simulink model "LKAS"  (R2018b)
settings: Solver=FixedStepDiscrete  StartTime=0.0  StopTime=10.0  FixedStep=0.01  RelTol=1e-3
InitFcn:
  | tmpVer = ver('MATLAB');
  | tmpVer = str2num(tmpVer.Version);
  | % -------------------------------------------------------------------
  | %  MATLAB file generated by Simulink.saveVars on 21-Nov-2019 10:06:14
  | %  MATLAB version: 7.13.0.564 (R2011b)
  | % -------------------------------------------------------------------
  | 
  | 
  | SInt16 = Simulink.AliasType;
  | SInt16.Description = 'Num';
  | if (tmpVer > 7.11)
  | 	SInt16.DataScope = 'Auto';
  | end
  | SInt16.HeaderFile = 'Rte_Type.h';
  | SInt16.BaseType = 'int16';
  | 
  | SInt32 = Simulink.AliasType;
  | SInt32.Description = 'Num';
  | if (tmpVer > 7.11)
  | 	SInt32.DataScope = 'Auto';
  | end
  | SInt32.HeaderFile = 'Rte_Type.h';
  | SInt32.BaseType = 'int32';
  | 
  | SInt8 = Simulink.AliasType;
  | SInt8.Description = 'Num';
  | if (tmpVer > 7.11)
  | 	SInt8.DataScope = 'Auto';
  | end
  | SInt8.HeaderFile = 'Rte_Type.h';
  | SInt8.BaseType = 'int8';
  | 
  | T_A_m2_1024_1_u32 = Simulink.NumericType;
  | T_A_m2_1024_1_u32.Description = 'm2 (square meters  (m2))';
  | if (tmpVer > 7.11)
  | 	T_A_m2_1024_1_u32.DataScope = 'Auto';
  | end
  | T_A_m2_1024_1_u32.HeaderFile = 'Rte_Type.h';
  | T_A_m2_1024_1_u32.DataTypeMode = 'Fixed-point: slope and bias scaling';
  | T_A_m2_1024_1_u32.SignednessBool = false;
  | T_A_m2_1024_1_u32.WordLength = 32;
  | T_A_m2_1024_1_u32.FixedExponent = -10;
  | T_A_m2_1024_1_u32.SlopeAdjustmentFactor = 1;
  | T_A_m2_1024_1_u32.Bias = 0;
  | T_A_m2_1024_1_u32.DataTypeOverride = 'Inherit';
  | T_A_m2_1024_1_u32.IsAlias = true;
  | 
  | T_A_m2_65536_1_u16 = Simulink.NumericType;
  | T_A_m2_65536_1_u16.Description = 'm2 (square meters  (m2))';
  | if (tmpVer > 7.11)
  | 	T_A_m2_65536_1_u16.DataScope = 'Auto';
  | end
  | T_A_m2_65536_1_u16.HeaderFile = 'Rte_Type.h';
  | T_A_m2_65536_1_u16.DataTypeMode = 'Fixed-point: slope and bias scaling';
  | T_A_m2_65536_1_u16.SignednessBool = false;
  | T_A_m2_65536_1_u16.WordLength = 16;
  | T_A_m2_65536_1_u16.FixedExponent = -16;
  | T_A_m2_65536_1_u16.SlopeAdjustmentFactor = 1;
  | T_A_m2_65536_1_u16.Bias = 0;
  | T_A_m2_65536_1_u16.DataTypeOverride = 'Inherit';
  | ... (+4598 lines)
StopFcn:
  | clear  T_A_m2_1024_1_u32 T_A_m2_65536_1_u16 T_A_m2_Float32 T_A_mm2_10_1_u16 T_A_mm2_4_1_s16 T_A_mm2_Float32 T_Cnt_Num_10_1_u32 T_Cnt_Num_1_1_s16 T_Cnt_Num_1_1_s32 T_Cnt_Num_1_1_s8 T_Cnt_Num_1_1_u16 T_Cnt_Num_1_1_u32 T_Cnt_Num_1_1_u8 T_E_J_1_1_s32 T_E_J_Float32 T_E_kJ_128_1_s32 T_E_kJ_Float32 T_E_kwh_10_1_u16 T_E_kwh_Float32 T_Epl_kwhpkm_100_1_u16 T_Epl_kwhpkm_Float32 T_F_N_1_1_s16 T_F_N_Float32 T_I_A_1000_1_u16 T_I_A_1048576_1_s32 T_I_A_2048_1_s16 T_I_A_32_1_s16 T_I_A_Float32 T_I_mA_1_1_s16 T_I_mA_32768_128_s16 T_I_mA_Float32 T_J_kgpm2_128_1_u16 T_J_kgpm2_Float32 T_K_NA_1000_1_s16 T_K_NA_100_1_s16 T_K_NA_100_1_u16 T_K_NA_1024_1_s16 T_K_NA_1024_1_u16 T_K_NA_128_1_s16 T_K_NA_128_1_u16 T_K_NA_128_1_u8 T_K_NA_16777216_1_u32 T_K_NA_16_1_s16 T_K_NA_16_1_u16 T_K_NA_16_1_u8 T_K_NA_1_16_u16 T_K_NA_1_1_s16 T_K_NA_1_1_u16 T_K_NA_1_1_u8 T_K_NA_32768_1_s16 T_K_NA_32768_1_u16 T_K_NA_32_1_s8 T_K_NA_4096_1_u16 T_K_NA_4194304_1_s32 T_K_NA_4194304_1_u16 T_K_NA_65536_1_s32 T_K_NA_65536_1_u16 T_K_NA_8192_1_s16 T_K_NA_8_1_s16 T_K_NA_Float32 T_M_Nm_16_1_s16 T_M_Nm_1_1_s16 T_M_Nm_32768_1_s16 T_M_Nm_32_1_s16 T_M_Nm_4_1_s16 T_M_Nm_512_1_s16 T_M_Nm_Float32 T_P_W_1_4_s16 T_P_W_1_8_s16 T_P_W_Float32 T_P_kW_128_1_s16 T_P_kW_1_8_s16 T_P_kW_8_1_s32 T_P_kW_Float32 T_Pct_pct_1024_1_s32 T_Pct_pct_1024_1_u32 T_Pct_pct_10_1_s16 T_Pct_pct_10_1_u32 T_Pct_pct_128_100_s8 T_Pct_pct_1_1_s16 T_Pct_pct_1_4_u8 T_Pct_pct_255_100_u16 T_Pct_pct_255_100_u8 T_Pct_pct_256_1_s16 T_Pct_pct_256_1_u16 T_Pct_pct_65535_100_u16 T_Pct_pct_Float32 T_R_ohm_1024_1_s16 T_R_ohm_32_1_s16 T_R_ohm_Float32 T_TK_K_16_1_s16 T_TK_K_Float32 T_T_degC_10_400_1_u16 T_T_degC_16_1_s16 T_T_degC_1_40_1_u8 T_T_degC_2_80_1_u8 T_T_degC_Float32 T_U_V_1000_1_u16 T_U_V_10_1_u8 T_U_V_200_1_u8 T_U_V_32_1_s16 T_U_V_4096_1_s16 T_U_V_512_1_s16 T_U_V_65535_8_u16 T_U_V_8192_1_u16 T_U_V_Float32 T_U_mV_1_1_s16 T_U_mV_256_20_u16 T_U_mV_Float32 T_V_l_256_1_s16 T_V_l_4096_1_s16 T_V_l_64_1_s16 T_V_l_65535_100_u16 T_V_l_Float32 T_V_ml_128_1_s16 T_V_ml_1_1_s16 T_V_ml_32768_1_s16 T_V_ml_Float32 T_V_ul_32_1_u16 T_V_ul_Float32 T_Vpl_clpkm_512_1_u16 T_Vpl_clpkm_Float32 T_a_kphps_16_1_s16 T_a_kphps_Float32 T_a_mps2_128_1_s16 T_a_mps2_Float32 T_c_MJpkg_256_1_s16 T_c_MJpkg_Float32 T_c_kJpgpK_1024_1_s16 T_c_kJpgpK_Float32 T_c_kJpkgpK_128_1_u16 T_c_kJpkgpK_Float32 T_chrg_Ah_1_1_s16 T_chrg_Ah_1_1_u16 T_chrg_Ah_1_1_u8 T_chrg_Ah_256_1_u16 T_chrg_Ah_4194304_1_s32 T_chrg_Ah_512_1_u16 T_chrg_Ah_8_1_u16 T_chrg_Ah_Float32 T_cmp_NA_100_1_s16 T_cmp_NA_128_1_s16 T_cmp_NA_16_1_s16 T_cmp_NA_32768_1_u16 T_cmp_NA_Float32 T_d2n_rpmps2_4_1_s16 T_d2n_rpmps2_Float32 T_dPct_pctps_16_1_s16 T_dPct_pctps_256_1_s16 T_dPct_pctps_Float32 T_dT_degCps_128_1_s16 T_dT_degCps_Float32 T_dV_lph_1_1_s16 T_dV_lph_Float32 T_dV_lpm_128_1_s16 T_dV_lpm_32_1_s16 T_dV_lpm_Float32 T_dV_lps_1024_1_u16 T_dV_lps_4_1_u16 T_dV_lps_Float32 T_dV_mlps_1024_1_s16 T_dV_mlps_Float32 T_d_BitField16 T_dm_gps_128_1_s16 T_dm_gps_128_1_u16 T_dm_gps_256_1_u16 T_dm_gps_Float32 T_dm_mgps_1_1_s16 T_dm_mgps_Float32 T_dn_rpmps_1_1_s16 T_dn_rpmps_2_1_s16 T_dn_rpmps_Float32 T_dp_Paps_1_1_s16 T_dp_Paps_Float32 T_dp_kPaps_1_1_s16 T_dp_kPaps_8_1_s16 T_dp_kPaps_Float32 T_dphi_degps_128_1_s16 T_dphi_degps_8_1_s16 T_dphi_degps_Float32 T_dr_ps_256_1_s16 T_dr_ps_Float32 T_drho_mgplps_1_2_s16 T_drho_mgplps_Float32 T_e_NA_1_1_u8 T_f_Hz_1_1_u16 T_f_Hz_1_1_u32 T_f_Hz_64_1_u16 T_f_Hz_8_1_s16 T_f_Hz_Float32 T_g_BitField32 T_l_km_16_1_s16 T_l_km_1_1_u16 T_l_km_1_1_u32 T_l_km_Float32 T_l_m_1024_1_s16 T_l_m_16_1_s16 T_l_m_1_1_u32 T_l_m_Float32 T_l_mm_16_1_s16 T_l_mm_1_1_u16 T_l_mm_4096_1_s16 T_l_mm_4_1_u8 T_l_mm_64_1_s16 T_l_mm_Float32 T_m_g_1_1_s16 T_m_g_2048_1_s16 T_m_g_32_1_u16 T_m_g_Float32 T_m_kg_1024_1_s16 T_m_kg_1_1_s16 T_m_kg_1_1_u32 T_m_kg_Float32 T_m_mg_128_1_s16 T_m_mg_32_1_s16 T_m_mg_Float32 T_n_rpm_1_1_s16 T_n_rpm_1_25_u8 T_n_rpm_256_50_u16 T_n_rpm_2_25_u8 T_n_rpm_4_1_u16 T_n_rpm_Float32 T_p_MPa_64_1_s16 T_p_MPa_Float32 T_p_Pa_1_1_s16 T_p_Pa_Float32 T_p_kPa_1_10_u16 T_p_kPa_1_1_s16 T_p_kPa_1_1_u8 T_p_kPa_256_1_u16 T_p_kPa_32_1_u16 T_p_kPa_64_1_s16 T_p_kPa_Float32 T_phi_deg_100_1_s16 T_phi_deg_1024_1_s16 T_phi_deg_128_1_s16 T_phi_deg_1_1_u8 T_phi_deg_256_1_s16 T_phi_deg_2_1_s8 T_phi_deg_32_1_s16 T_phi_deg_512_6_s32 T_phi_deg_Float32 T_phi_rad_2048_1_s16 T_phi_rad_Float32 T_r_NA_1024_1_s16 T_r_NA_1024_1_u16 T_r_NA_16384_1_s16 T_r_NA_16_1_s16 T_r_NA_256_1_s8 T_r_NA_256_1_u16 T_r_NA_32768_1_u16 T_r_NA_32_1_u16 T_r_NA_4096_1_s16 T_r_NA_65535_2_u16 T_r_NA_8192_1_u16 T_r_NA_Float32 T_rho_gpl_8192_1_s16 T_rho_gpl_Float32 T_rho_kgpm3_16_1_s16 T_rho_kgpm3_Float32 T_rho_mgpl_1_1_s16 T_rho_mgpl_64_1_s16 T_rho_mgpl_Float32 T_t_hour_1_1_s16 T_t_hour_Float32 T_t_m_1_1_u16 T_t_m_Float32 T_t_ms_1_1_s16 T_t_ms_1_1_u16 T_t_ms_1_1_u32 T_t_ms_4096_1_s16 T_t_ms_64_1_s16 T_t_ms_Float32 T_t_s_1000_1_s16 T_t_s_100_1_s16 T_t_s_10_1_s16 T_t_s_10_1_u16 T_t_s_1_1_s16 T_t_s_1_1_u16 T_t_s_1_1_u32 T_t_s_Float32 T_t_us_10_1_u32 T_t_us_1_1_s16 T_t_us_1_1_u32 T_t_us_1_4_u16 T_t_us_Float32 T_v_kph_1_1_u8 T_v_kph_64_1_s16 T_v_kph_64_1_u16 T_v_kph_Float32 T_v_mps_256_1_s16 T_v_mps_Float32 T_w_radps_32_1_s16 T_w_radps_Float32 T_y_BitField8 T_y_BitFieldDiagProgress T_y_BitFieldDiagStatus T_y_NA_1_1_u8 SInt16 SInt32 SInt8 T_BOOLEAN UInt16 UInt32 UInt8 s16 s32 s8 u16 u32 u8
model workspace (MAT data in the model file):
  MCOS : class17 (value not decoded)
  MCOS : class17 (value not decoded)
  MCOS : class17 (value not decoded)
  MCOS : class17 (value not decoded)
  MCOS : class17 (value not decoded)
  MCOS : class17 (value not decoded)
  MCOS : class17 (value not decoded)
  MCOS : class17 (value not decoded)
  MCOS : class17 (value not decoded)
  MCOS : class17 (value not decoded)
  MCOS : class17 (value not decoded)
  MCOS : class17 (value not decoded)
  MCOS : class17 (value not decoded)
  MCOS : class17 (value not decoded)
  MCOS : class17 (value not decoded)
  MCOS : class17 (value not decoded)
  MCOS : class17 (value not decoded)
  MCOS : class17 (value not decoded)
  MCOS : class17 (value not decoded)
  MCOS : class17 (value not decoded)
  MCOS : class17 (value not decoded)
  MCOS : class17 (value not decoded)
  MCOS : class17 (value not decoded)
  MCOS : class17 (value not decoded)
  MCOS : class17 (value not decoded)
  MCOS : class17 (value not decoded)
  MCOS : class17 (value not decoded)
  MCOS : class17 (value not decoded)
  MCOS : class17 (value not decoded)
  MCOS : class17 (value not decoded)
  MCOS : class17 (value not decoded)
  MCOS : class17 (value not decoded)
  MCOS : class17 (value not decoded)
  MCOS : class17 (value not decoded)
  MCOS : class17 (value not decoded)
  MCOS : class17 (value not decoded)
  MCOS : class17 (value not decoded)
  MCOS : class17 (value not decoded)
  MCOS : class17 (value not decoded)
  MCOS : class17 (value not decoded)
  MCOS : class17 (value not decoded)
  MCOS : class17 (value not decoded)
  MCOS : class17 (value not decoded)
  MCOS : class17 (value not decoded)
  MCOS : class17 (value not decoded)
  MCOS : class17 (value not decoded)
  MCOS : class17 (value not decoded)
  MCOS : class17 (value not decoded)
  MCOS : class17 (value not decoded)
  MCOS : class17 (value not decoded)
  MCOS : class17 (value not decoded)
  MCOS : class17 (value not decoded)
  MCOS : class17 (value not decoded)
  MCOS : class17 (value not decoded)
  MCOS : class17 (value not decoded)
  MCOS : class17 (value not decoded)
  MCOS : class17 (value not decoded)
  MCOS : class17 (value not decoded)
  MCOS : class17 (value not decoded)
  MCOS : class17 (value not decoded)
  MCOS : class17 (value not decoded)
  MCOS : class17 (value not decoded)
  MCOS : class17 (value not decoded)
  MCOS : class17 (value not decoded)
  MCOS : class17 (value not decoded)
  MCOS : class17 (value not decoded)
  MCOS : class17 (value not decoded)
  MCOS : class17 (value not decoded)
  MCOS : class17 (value not decoded)
  MCOS : class17 (value not decoded)
  MCOS : class17 (value not decoded)
  MCOS : class17 (value not decoded)
  MCOS : class17 (value not decoded)
  MCOS : class17 (value not decoded)
  MCOS : class17 (value not decoded)
  MCOS : class17 (value not decoded)
  MCOS : class17 (value not decoded)
  MCOS : class17 (value not decoded)
  MCOS : class17 (value not decoded)
  MCOS : class17 (value not decoded)
  MCOS : class17 (value not decoded)
  MCOS : class17 (value not decoded)
  MCOS : class17 (value not decoded)
  MCOS : class17 (value not decoded)
  MCOS : class17 (value not decoded)
  MCOS : class17 (value not decoded)
  MCOS : class17 (value not decoded)
  MCOS : class17 (value not decoded)
  MCOS : class17 (value not decoded)
undefined symbols (not defined in the file): LKA_CarWidth, LKA_SampleTime, LKA_StrRatio_C, LKA_Veh2CamL_C, LKA_Veh2CamW_C, LKA_WhlBaseL_C, LL_CompSWA_C, LL_CrvtPrvwT_C, LL_DesDvt_C, LL_DvtComp_C, LL_DvtPrvwT_C, LL_DvtSpdDet_vDvtSpdMin_C, LL_HdAgExT_C, LL_HdAgPrvwT_C, LL_LAccMax_C, LL_LAccRMax_C, LL_LDW_EarliestWarnLine_C, LL_LDW_LatestWarnLine_C, LL_LDWS_SUPPRESS_HEADING, LL_LFClb_TFC_DiffCtlBalance, LL_LFClb_TFC_DiffCtrlMaxSWA, LL_LFClb_TFC_DiffCtrlRatio, LL_LFClb_TFC_facmGainLutGain1_C, LL_LFClb_TFC_facmGainLutGain2_C, LL_LFClb_TFC_facmIntegRatio, LL_LFClb_TFC_facmKlat_C, LL_LFClb_TFC_FfCtlRatio_C, LL_LFClb_TFC_phiIntegCtlMaxSWA_C, LL_LFClb_TFC_tiKlatPrvwT_C, LL_LFClb_TFC_vGainLutVehSpdLwr_C, LL_LFClb_TFC_vGainLutVehSpdUpr_C, LL_LKA_EarliestWarnLine_C, LL_LKA_LatestWarnLine_C, LL_LKAExPrcs_ExitC0Dvt, LL_LKAExPrcs_ExitC0Swt, LL_LKAExPrcs_tiExitTime1, LL_LKAExPrcs_tiExitTime2, LL_LKAExPrcs_tiExitTime3, LL_LKAS_OUT_OF_CONTROL_LAT_VEL, LL_LKAS_OUT_OF_CONTROL_TTLC, LL_LKASWASyn_M0, LL_LKASWASyn_M1, LL_LKASWASyn_M2, LL_LKASWASyn_M3K, LL_LKASWASyn_SWAaddMax, LL_LKASWASyn_T2, LL_LKASWASyn_tiTrqSwaRtTime, LL_LKASWASyn_tiTrqSwaTime, LL_LKASWASyn_TrqMax, LL_LKASWASyn_TrqSwaAddSwt, LL_LKASWASyn_TrqSwaRateDiff, LL_LSpdCompT_C, LL_lStpLngth_C, LL_MAX_DELAY_EPSSTAR_TIME, LL_MAX_DRIVER_TORQUE_DISABLE, LL_MAX_DRIVER_TORQUE_ENABLE, LL_MAX_LANE_WIDTH_DISABLE, LL_MAX_LANE_WIDTH_ENABLE, LL_MAX_LAT_ACC_DISABLE, LL_MAX_LAT_ACC_ENABLE ... (+29)
libraries: simulink x190, dspstat3 x3, simulink_extras x1
(part 14 of 19)

== system LKAS/LKAS/LL/LLOn/LKA/LKA Motion Planning (LKAMP) /LKA Motion Planning Calculation (LKAMPCal)/Time Division (TDiv)/if action 1 ==
  In1 : Inport
  Action Port : ActionPort  InitializeStates=reset  ActionType=else
  Out1 : Outport
  wires:
  In1/1 -> Out1/1

== system LKAS/LKAS/LL/LLOn/LKA/LKA Motion Planning (LKAMP) /LKA Motion Planning Calculation (LKAMPCal)/Time Division (TDiv)/if action 2 ==
  Action Port : ActionPort  InitializeStates=reset  ActionType=then
  Constant : Constant  Value=0  OutDataTypeStr=uint16
  Out1 : Outport
  wires:
  Constant/1 -> Out1/1  "ModeFlg"

== system LKAS/LKAS/LL/LLOn/LKA/LKA Motion Planning (LKAMP) /LKA Motion Planning Calculation (LKAMPCal)/Time Division (TDiv)1/if action 3 ==
  In1 : Inport
  Action Port : ActionPort  InitializeStates=reset  ActionType=else
  Out1 : Outport
  wires:
  In1/1 -> Out1/1

== system LKAS/LKAS/LL/LLOn/LKA/LKA Motion Planning (LKAMP) /LKA Motion Planning Calculation (LKAMPCal)/Time Division (TDiv)1/if action 4 ==
  Action Port : ActionPort  InitializeStates=reset  ActionType=then
  Constant : Constant  Value=0  OutDataTypeStr=single
  Out1 : Outport
  wires:
  Constant/1 -> Out1/1  "ModeFlg"

== system LKAS/LKAS/LL/LLOn/LKA/LKA Motion Planning (LKAMP) /LKA Motion Planning Calculation (LKAMPCal)/Time Division (TDiv)2/if action 3 ==
  In1 : Inport
  Action Port : ActionPort  InitializeStates=reset  ActionType=else
  Out1 : Outport
  wires:
  In1/1 -> Out1/1

== system LKAS/LKAS/LL/LLOn/LKA/LKA Motion Planning (LKAMP) /LKA Motion Planning Calculation (LKAMPCal)/Time Division (TDiv)2/if action 4 ==
  Action Port : ActionPort  InitializeStates=reset  ActionType=then
  Constant : Constant  Value=0  OutDataTypeStr=single
  Out1 : Outport
  wires:
  Constant/1 -> Out1/1  "ModeFlg"

== system LKAS/LKAS/LL/LLOn/LKA/LKA Motion Planning (LKAMP) /LKA Motion Planning Calculation (LKAMPCal)/Time Division (TDiv)3/if action 3 ==
  In1 : Inport
  Action Port : ActionPort  InitializeStates=reset  ActionType=else
  Out1 : Outport
  wires:
  In1/1 -> Out1/1

== system LKAS/LKAS/LL/LLOn/LKA/LKA Motion Planning (LKAMP) /LKA Motion Planning Calculation (LKAMPCal)/Time Division (TDiv)3/if action 4 ==
  Action Port : ActionPort  InitializeStates=reset  ActionType=then
  Constant : Constant  Value=0  OutDataTypeStr=single
  Out1 : Outport
  wires:
  Constant/1 -> Out1/1  "ModeFlg"

== system LKAS/LKAS/LL/LLOn/LKA/LKA Motion Planning (LKAMP) /LKA Motion Planning Calculation (LKAMPCal)/Time Division (TDiv)4/if action 3 ==
  In1 : Inport
  Action Port : ActionPort  InitializeStates=reset  ActionType=else
  Out1 : Outport
  wires:
  In1/1 -> Out1/1

== system LKAS/LKAS/LL/LLOn/LKA/LKA Motion Planning (LKAMP) /LKA Motion Planning Calculation (LKAMPCal)/Time Division (TDiv)4/if action 4 ==
  Action Port : ActionPort  InitializeStates=reset  ActionType=then
  Constant : Constant  Value=0  OutDataTypeStr=single
  Out1 : Outport
  wires:
  Constant/1 -> Out1/1  "ModeFlg"

== system LKAS/LKAS/LL/LLOn/LKA/LKA Motion Planning (LKAMP) /Motion Planning Input Processing (MPInP)/Lane Information Selection (LaneInfoSel)/If Action Subsystem1 ==
  In1 : Inport
  Action Port : ActionPort  InitializeStates=reset  ActionType=elseif
  Out1 : Outport
  wires:
  In1/1 -> Out1/1

== system LKAS/LKAS/LL/LLOn/LKA/LKA Motion Planning (LKAMP) /Motion Planning Input Processing (MPInP)/Lane Information Selection (LaneInfoSel)/If Action Subsystem2 ==
  In1 : Inport
  Action Port : ActionPort  InitializeStates=reset  ActionType=then
  Out1 : Outport
  wires:
  In1/1 -> Out1/1

== system LKAS/LKAS/LL/LLOn/LKA/LKA Motion Planning (LKAMP) /Motion Planning Input Processing (MPInP)/Lane Information Selection (LaneInfoSel)/If Action Subsystem3 ==
  Action Port : ActionPort  InitializeStates=reset  ActionType=else
  Constant : Constant  Value=0  OutDataTypeStr=single
  Out1 : Outport
  wires:
  Constant/1 -> Out1/1

== system LKAS/LKAS/LL/LLOn/LKA/LKA Motion Planning (LKAMP) /Motion Planning Input Processing (MPInP)/Signal Latching2/if action  ==
  In : Inport
  Action Port : ActionPort  InitializeStates=reset  ActionType=then
  Out : Outport
  wires:
  In/1 -> Out/1

== system LKAS/LKAS/LL/LLOn/LKA/LKA Motion Planning (LKAMP) /Motion Planning Input Processing (MPInP)/Signal Latching3/if action  ==
  In : Inport
  Action Port : ActionPort  InitializeStates=reset  ActionType=then
  Out : Outport
  wires:
  In/1 -> Out/1

== system LKAS/LKAS/LL/LLOn/LKA/LKA Motion Planning (LKAMP) /Motion Planning Input Processing (MPInP)/Signal Latching4/if action  ==
  In : Inport
  Action Port : ActionPort  InitializeStates=reset  ActionType=then
  Out : Outport
  wires:
  In/1 -> Out/1

== system LKAS/LKAS/LL/LLOn/LKA/LKA Motion Planning (LKAMP) /Motion Planning Input Processing (MPInP)/Signal Latching5/if action  ==
  In : Inport
  Action Port : ActionPort  InitializeStates=reset  ActionType=then
  Out : Outport
  wires:
  In/1 -> Out/1

== system LKAS/LKAS/LL/LLOn/LKA/LKA Motion Planning (LKAMP) /Motion Planning Input Processing (MPInP)/Signal Latching6/if action  ==
  In : Inport
  Action Port : ActionPort  InitializeStates=reset  ActionType=then
  Out : Outport
  wires:
  In/1 -> Out/1

== system LKAS/LKAS/LL/LLOn/LKA/LKA Motion Planning (LKAMP) /Motion Planning Input Processing (MPInP)/Signal Latching7/if action  ==
  In : Inport
  Action Port : ActionPort  InitializeStates=reset  ActionType=then
  Out : Outport
  wires:
  In/1 -> Out/1

== system LKAS/LKAS/LL/LLOn/LKA/LKA Motion Planning (LKAMP) /Motion Planning Input Processing (MPInP)/Subsystem/If Action Subsystem1 ==
  Action Port : ActionPort  InitializeStates=reset  ActionType=elseif
  Constant : Constant  OutDataTypeStr=single
  Out1 : Outport
  wires:
  Constant/1 -> Out1/1

== system LKAS/LKAS/LL/LLOn/LKA/LKA Motion Planning (LKAMP) /Motion Planning Input Processing (MPInP)/Subsystem/If Action Subsystem2 ==
  Action Port : ActionPort  InitializeStates=reset  ActionType=then
  Constant : Constant  Value=-1  OutDataTypeStr=single
  Out1 : Outport
  wires:
  Constant/1 -> Out1/1

== system LKAS/LKAS/LL/LLOn/LKA/LKA Motion Planning (LKAMP) /Motion Planning Input Processing (MPInP)/Subsystem/If Action Subsystem3 ==
  Action Port : ActionPort  InitializeStates=reset  ActionType=else
  Constant : Constant  Value=0  OutDataTypeStr=single
  Out1 : Outport
  wires:
  Constant/1 -> Out1/1

== system LKAS/LKAS/LL/LLOn/LKA/LKA Motion Planning (LKAMP) /Switching Condition (SwtCon)/Ending Heading Angle Determination (EndHdAgDet)/Lateral Speed Compensation (LSpdComp) ==
  LSpdComp_vVehSpd : Inport
  LSpdComp_stLKAFlg : Inport  Port=2
  LSpdComp_crPrvwCrvt : Inport  Port=3
  LSpdComp_tiLSpdCompT_C : Inport  Port=4
  Abs : Abs
  Abs1 : Abs
  Compare To Zero : simulink/Logic and Bit Operations/Compare To Zero  relop=<=  OutDataTypeStr=boolean
  Data Type Conversion : DataTypeConversion  OutDataTypeStr=uint8
  Divide : Product  Inputs=***
  If : If  NumInputs=2  IfExpression=u1==1&u2==0  ElseIfExpressions=u1==2&u2==1
  If Action Subsystem : Subsystem  TreatAsAtomicUnit=on
  If Action Subsystem2 : Subsystem  TreatAsAtomicUnit=on
  If Action Subsystem4 : Subsystem  TreatAsAtomicUnit=on
  Merge : Merge  Inputs=3
  LSpdComp_phiLSpdComp : Outport
  wires:
  Divide/1 -> Abs/1, Abs1/1
  LSpdComp_tiLSpdCompT_C/1 -> Divide/3
  LSpdComp_vVehSpd/1 -> Divide/2
  Abs1/1 -> If Action Subsystem4/1(In1)
  Abs/1 -> If Action Subsystem/1(In1)
  If/2 -> If Action Subsystem4/Action
  If Action Subsystem4/1(Out1) -> Merge/2
  If Action Subsystem2/1(Out1) -> Merge/3
  Data Type Conversion/1 -> If/2
  Compare To Zero/1 -> Data Type Conversion/1
  LSpdComp_crPrvwCrvt/1 -> Compare To Zero/1, Divide/1
  If/1 -> If Action Subsystem/Action
  If Action Subsystem/1(Out1) -> Merge/1
  If/3 -> If Action Subsystem2/Action
  Merge/1 -> LSpdComp_phiLSpdComp/1
  LSpdComp_stLKAFlg/1 -> If/1

== system LKAS/LKAS/LL/LLOn/LKA/LKA Motion Planning (LKAMP) /Switching Condition (SwtCon)/Signal Latching/if action  ==
  In : Inport
  Action Port : ActionPort  InitializeStates=reset  ActionType=then
  Out : Outport
  wires:
  In/1 -> Out/1

== system LKAS/LKAS/LL/LLOn/LKA/Lane Following (LF)/Trajectory Following Control (TFC)/Feedback Control (FbCtl)/Average Filter (AvrgFlt) ==
  In : Inport
  PtsNum : Inport  Port=2
  Add1 : Sum
  Add2 : Sum  Inputs=-+
  Constant : Constant  OutDataTypeStr=single
  Constant1 : Constant  OutDataTypeStr=single
  Divide : Product  Inputs=**
  Divide1 : Product  Inputs=**
  Divide2 : Product  Inputs=*/
  Memory : Memory  InheritSampleTime=on
  Saturation : Saturate  UpperLimit=10000  LowerLimit=1  OutDataTypeStr=single
  Out : Outport
  wires:
  Constant1/1 -> Divide2/1
  Saturation/1 -> Divide2/2
  Memory/1 -> Divide1/2
  Divide2/1 -> Divide/2, Add2/1
  Add1/1 -> Memory/1, Out/1
  Divide1/1 -> Add1/2
  Add2/1 -> Divide1/1
  Constant/1 -> Add2/2
  Divide/1 -> Add1/1
  PtsNum/1 -> Saturation/1
  In/1 -> Divide/1

== system LKAS/LKAS/LL/LLOn/LKA/Lane Following (LF)/Trajectory Following Control (TFC)/Feedback Control (FbCtl)/Subsystem ==
  L0C0 : Inport
  R0C0 : Inport  Port=2
  FbCtl_DiffCtlRatio : Inport  Port=3
  FbCtl_DiffCtlBalance : Inport  Port=4
  Abs5 : Abs
  Abs7 : Abs
  Add1 : Sum
  Add2 : Sum
  Add5 : Sum
  Add6 : Sum  Inputs=++-
  Constant2 : Constant  OutDataTypeStr=single
  Constant3 : Constant  OutDataTypeStr=single
  Divide1 : Product  Inputs=*/
  Divide2 : Product  Inputs=**
  Divide4 : Product  Inputs=*/
  Divide5 : Product  Inputs=**
  If : If  IfExpression=u1 == 1  ElseIfExpressions=u1 == 2
  If Action Subsystem : Subsystem  TreatAsAtomicUnit=on
  If Action Subsystem1 : Subsystem  TreatAsAtomicUnit=on
  If Action Subsystem2 : Subsystem  TreatAsAtomicUnit=on
  Merge : Merge  Inputs=3
  Saturation : Saturate  UpperLimit=2  LowerLimit=-2
  Saturation1 : Saturate  UpperLimit=1000  LowerLimit=0
  Signal Latching2 : Subsystem  mask(Signal Latching:){LatchTime=1}
      mask prompts: LatchTime "Latch time(-):"
      mask help:
      | If the latch time is not reached, the input signal will just go through the block. If the latch time is reached, the output will be held and do not change again. The latch time is described with the number of the sampling time.
      | ----vcdc.ascl@jlu 19-01-15
  Unary Minus : UnaryMinus
  D : Outport
  wires:
  Abs5/1 -> Add6/1
  Constant3/1 -> Add5/1
  Add2/1 -> Saturation/1
  L0C0/1 -> Add2/1, Abs5/1
  FbCtl_DiffCtlRatio/1 -> Divide2/2, Divide5/2, If Action Subsystem2/1(In1)
  Abs7/1 -> Add6/2
  Divide4/1 -> Add5/2
  R0C0/1 -> Abs7/1, Add2/2
  Add6/1 -> Divide1/2, Divide4/2
  FbCtl_DiffCtlBalance/1 -> Add6/3
  Add5/1 -> Divide5/1
  Saturation1/1 -> D/1  "D"
  [ActFlg] -> Signal Latching2/1(In)
  If/1 -> If Action Subsystem/Action
  Signal Latching2/1(Out) -> If/1  "ActFlg"
  Add1/1 -> Divide2/1
  Divide1/1 -> Add1/2
  Constant2/1 -> Add1/1
  Unary Minus/1 -> Divide1/1
  If/2 -> If Action Subsystem1/Action
  If/3 -> If Action Subsystem2/Action
  If Action Subsystem/1(Out1) -> Merge/1
  If Action Subsystem1/1(Out1) -> Merge/2
  If Action Subsystem2/1(Out1) -> Merge/3
  Divide5/1 -> If Action Subsystem1/1(In1)
  Divide2/1 -> If Action Subsystem/1(In1)
  Saturation/1 -> Divide4/1, Unary Minus/1
  Merge/1 -> Saturation1/1

== system LKAS/LKAS/LL/LLOn/LKA/Lane Following (LF)/Trajectory Following Control (TFC)/Feedback Control (FbCtl)/Time ==
  Add2 : Sum  OutDataTypeStr=single
  Memory3 : Memory  InheritSampleTime=on
  Saturation : Saturate  UpperLimit=50  LowerLimit=0
  Out1 : Outport
  wires:
  Add2/1 -> Saturation/1
  Memory3/1 -> Add2/2
  Saturation/1 -> Out1/1, Memory3/1
  [LKA_SampleTime] -> Add2/1

== system LKAS/LKAS/LL/LLOn/LKA/Plan To LaneFollowing (PTLF)/InsideJudge1/If Action Subsystem/If Action Subsystem ==
  T1 : Inport
  Plan : Inport  Port=2
  Enable : EnablePort
  Signal Latching : Subsystem  mask(Signal Latching:){LatchTime=1}
      mask prompts: LatchTime "Latch time(-):"
      mask help:
      | If the latch time is not reached, the input signal will just go through the block. If the latch time is reached, the output will be held and do not change again. The latch time is described with the number of the sampling time.
      | ----vcdc.ascl@jlu 19-01-15
  Signal Latching1 : Subsystem  mask(Signal Latching:){LatchTime=1}
      mask prompts: LatchTime "Latch time(-):"
      mask help:
      | If the latch time is not reached, the input signal will just go through the block. If the latch time is reached, the output will be held and do not change again. The latch time is described with the number of the sampling time.
      | ----vcdc.ascl@jlu 19-01-15
  T1_1 : Outport
  Plan_1 : Outport  Port=2
  wires:
  Signal Latching/1(Out) -> T1_1/1
  Signal Latching1/1(Out) -> Plan_1/1
  T1/1 -> Signal Latching/1(In)
  Plan/1 -> Signal Latching1/1(In)

== system LKAS/LKAS/LL/LLOn/LKA/Plan To LaneFollowing (PTLF)/InsideJudge1/If Action Subsystem/If Action Subsystem2 ==
  T1 : Inport
  Plan : Inport  Port=2
  T1_1 : Outport
  Plan_1 : Outport  Port=2
  wires:
  T1/1 -> T1_1/1
  Plan/1 -> Plan_1/1

== system LKAS/LKAS/LL/LLOn/LKA/Plan To LaneFollowing (PTLF)/InsideJudge1/If Action Subsystem1/If Action Subsystem ==
  T1 : Inport
  Plan : Inport  Port=2
  Enable : EnablePort
  Signal Latching : Subsystem  mask(Signal Latching:){LatchTime=1}
      mask prompts: LatchTime "Latch time(-):"
      mask help:
      | If the latch time is not reached, the input signal will just go through the block. If the latch time is reached, the output will be held and do not change again. The latch time is described with the number of the sampling time.
      | ----vcdc.ascl@jlu 19-01-15
  Signal Latching1 : Subsystem  mask(Signal Latching:){LatchTime=1}
      mask prompts: LatchTime "Latch time(-):"
      mask help:
      | If the latch time is not reached, the input signal will just go through the block. If the latch time is reached, the output will be held and do not change again. The latch time is described with the number of the sampling time.
      | ----vcdc.ascl@jlu 19-01-15
  T1_1 : Outport
  Plan_1 : Outport  Port=2
  wires:
  Signal Latching/1(Out) -> T1_1/1
  Signal Latching1/1(Out) -> Plan_1/1
  T1/1 -> Signal Latching/1(In)
  Plan/1 -> Signal Latching1/1(In)

== system LKAS/LKAS/LL/LLOn/LKA/Plan To LaneFollowing (PTLF)/InsideJudge1/If Action Subsystem1/If Action Subsystem2 ==
  T1 : Inport
  Plan : Inport  Port=2
  T1_1 : Outport
  Plan_1 : Outport  Port=2
  wires:
  T1/1 -> T1_1/1
  Plan/1 -> Plan_1/1

== system LKAS/LKAS/LL/LLOn/LL State Determination (LLStateDet)/LL State Machine Conditions (LLSMCon)/Activation Condition (ActvC)/Activation Condition Synthesis (ActvCSyn)/Default Flag (DflFlg) ==
  Action Port : ActionPort  InitializeStates=reset  ActionType=else
  Constant : Constant  Value=0  OutDataTypeStr=uint8  SampleTime=-1
  Out : Outport
  wires:
  Constant/1 -> Out/1

== system LKAS/LKAS/LL/LLOn/LL State Determination (LLStateDet)/LL State Machine Conditions (LLSMCon)/Activation Condition (ActvC)/Activation Condition Synthesis (ActvCSyn)/Default Flag (DflFlg)1 ==
  Action Port : ActionPort  InitializeStates=reset  ActionType=else
  Constant : Constant  Value=0  OutDataTypeStr=uint8  SampleTime=-1
  Out : Outport
  wires:
  Constant/1 -> Out/1

== system LKAS/LKAS/LL/LLOn/LL State Determination (LLStateDet)/LL State Machine Conditions (LLSMCon)/Activation Condition (ActvC)/Activation Condition Synthesis (ActvCSyn)/LDW Left Active Flag (LDWLftActvFlg) ==
  Action Port : ActionPort  InitializeStates=reset  ActionType=then
  Constant : Constant  OutDataTypeStr=uint8  SampleTime=-1
  Out : Outport
  wires:
  Constant/1 -> Out/1

== system LKAS/LKAS/LL/LLOn/LL State Determination (LLStateDet)/LL State Machine Conditions (LLSMCon)/Activation Condition (ActvC)/Activation Condition Synthesis (ActvCSyn)/LDW Right Active Flag (LDWRgtActvFlg) ==
  Action Port : ActionPort  InitializeStates=reset  ActionType=elseif
  Constant : Constant  Value=2  OutDataTypeStr=uint8  SampleTime=-1
  Out : Outport
  wires:
  Constant/1 -> Out/1

== system LKAS/LKAS/LL/LLOn/LL State Determination (LLStateDet)/LL State Machine Conditions (LLSMCon)/Activation Condition (ActvC)/Activation Condition Synthesis (ActvCSyn)/LKA Left Active Flag (LKALftActvFlg)1 ==
  Action Port : ActionPort  InitializeStates=reset  ActionType=then
  Constant : Constant  OutDataTypeStr=uint8  SampleTime=-1
  Out : Outport
  wires:
  Constant/1 -> Out/1

== system LKAS/LKAS/LL/LLOn/LL State Determination (LLStateDet)/LL State Machine Conditions (LLSMCon)/Activation Condition (ActvC)/Activation Condition Synthesis (ActvCSyn)/LKA Right Active Flag (LKARgtActvFlg)1 ==
  Action Port : ActionPort  InitializeStates=reset  ActionType=elseif
  Constant : Constant  Value=2  OutDataTypeStr=uint8  SampleTime=-1
  Out : Outport
  wires:
  Constant/1 -> Out/1

== system LKAS/LKAS/LL/LLOn/LL State Determination (LLStateDet)/LL State Machine Conditions (LLSMCon)/Activation Condition (ActvC)/Deviation Threshold Condition (DvtThresCon)/Active Lane Calculation (ActLanCalc) ==
  ActLanCalc_bsL0Info : Inport
  ActLanCalc_bsR0Info : Inport  Port=2
  ActLanCalc_ActvCClb : Inport  Port=3
  Abs2 : Abs
  Abs3 : Abs
  Add1 : Sum
  Add2 : Sum  Inputs=+-
  Bus Creator : BusCreator  Inputs=7
  Bus Selector1 : BusSelector  OutputSignals=R0_C0
  Bus Selector2 : BusSelector  OutputSignals=L0_C0
  Bus Selector3 : BusSelector  OutputSignals=LL_ThresDet_lDvtThresLwrLDW,LL_ThresDet_lDvtThresUprLDW,LL_ThresDet_tiTTLCThresLDW,LL_ThresDet_lDvtThresLwrLKA,LL_ThresDet_lDvtThresUprLKA,LL_ThresDet_tiTTLCThresLKA,LL_DvtSpdDet_vDvtSpdMin_C
  Constant1 : Constant  Value=0.6  OutDataTypeStr=single
  Constant2 : Constant  Value=0.3  OutDataTypeStr=single
  Divide : Product  Inputs=*/
  Divide{1..6} (6 alike) : Product  Inputs=**
  Gain : Gain  Gain=0.25
  Saturation1 : Saturate  UpperLimit=5.5  LowerLimit=2.4
  Saturation2 : Saturate  UpperLimit=0.3  LowerLimit=0
  ActLanCalc_ActvCClbOut : Outport
  wires:
  Bus Selector3/7 -> Bus Creator/7  "<LL_DvtSpdDet_vDvtSpdMin_C>"
  Bus Creator/1 -> ActLanCalc_ActvCClbOut/1
  Divide6/1 -> Bus Creator/6  "LL_ThresDet_tiTTLCThresLKA"
  Divide5/1 -> Bus Creator/5  "LL_ThresDet_lDvtThresUprLKA"
  Divide4/1 -> Bus Creator/4  "LL_ThresDet_lDvtThresLwrLKA"
  Divide3/1 -> Bus Creator/3  "LL_ThresDet_tiTTLCThresLDW"
  Divide2/1 -> Bus Creator/2  "LL_ThresDet_lDvtThresUprLDW"
  Divide1/1 -> Bus Creator/1  "LL_ThresDet_lDvtThresLwrLDW"
  Divide/1 -> Divide1/1, Divide3/1, Divide4/1, Divide5/1, Divide6/1, Divide2/1
  Bus Selector3/6 -> Divide6/2  "<LL_ThresDet_tiTTLCThresLKA>"
  Bus Selector3/5 -> Divide5/2  "<LL_ThresDet_lDvtThresUprLKA>"
  Bus Selector3/4 -> Divide4/2  "<LL_ThresDet_lDvtThresLwrLKA>"
  Bus Selector3/3 -> Divide3/2  "<LL_ThresDet_tiTTLCThresLDW>"
  Saturation2/1 -> Divide/1
  Constant2/1 -> Divide/2
  Bus Selector3/2 -> Divide2/2  "<LL_ThresDet_lDvtThresUprLDW>"
  Bus Selector3/1 -> Divide1/2  "<LL_ThresDet_lDvtThresLwrLDW>"
  Add2/1 -> Saturation2/1
  Abs2/1 -> Add1/1
  Saturation1/1 -> Gain/1
  Constant1/1 -> Add2/2
  Abs3/1 -> Add1/2
  Add1/1 -> Saturation1/1
  Gain/1 -> Add2/1
  ActLanCalc_ActvCClb/1 -> Bus Selector3/1
  Bus Selector1/1 -> Abs3/1  "<R0_C0>"
  Bus Selector2/1 -> Abs2/1  "<L0_C0>"
  ActLanCalc_bsR0Info/1 -> Bus Selector1/1
  ActLanCalc_bsL0Info/1 -> Bus Selector2/1

== system LKAS/LKAS/LL/LLOn/LL State Determination (LLStateDet)/LL State Machine Conditions (LLSMCon)/Activation Condition (ActvC)/Deviation Threshold Condition (DvtThresCon)/Deviation Calculation (DvtCalc) ==
  DvtCalc_bsL0Info : Inport
  DvtCalc_bsR0Info : Inport  Port=2
  Bus Selector1 : BusSelector  OutputSignals=R0_C0,R0_C1
  Bus Selector2 : BusSelector  OutputSignals=L0_C0,L0_C1
  Bus Selector3 : BusSelector  OutputSignals=EnaCClb.LL_DvtComp_C
  Left Front Conner Deviation Calculation (LFCDvtCalc) : Subsystem
  Right Front Conner Deviation Calculation (RFCDvtCalc) : Subsystem
  Saturation : Saturate  UpperLimit=2  LowerLimit=-4
  Saturation1 : Saturate  UpperLimit=0.2  LowerLimit=-0.2
  Saturation2 : Saturate  UpperLimit=4  LowerLimit=-2
  Saturation3 : Saturate  UpperLimit=0.2  LowerLimit=-0.2
  Saturation4 : Saturate  UpperLimit=0.1  LowerLimit=-0.1
  DvtCalc_lLftDvt : Outport
  DvtCalc_lRgtDvt : Outport  Port=2
  wires:
  DvtCalc_bsL0Info/1 -> Bus Selector2/1
  DvtCalc_bsR0Info/1 -> Bus Selector1/1
  Left Front Conner Deviation Calculation (LFCDvtCalc)/1(DvtCalc_lLftDvt) -> DvtCalc_lLftDvt/1
  Right Front Conner Deviation Calculation (RFCDvtCalc)/1(DvtCalc_lRgtDvt) -> DvtCalc_lRgtDvt/1
  Bus Selector2/1 -> Saturation/1  "<L0_C0>"
  Bus Selector2/2 -> Saturation1/1  "<L0_C1>"
  Bus Selector1/1 -> Saturation2/1  "<R0_C0>"
  Bus Selector1/2 -> Saturation3/1  "<R0_C1>"
  Bus Selector3/1 -> Saturation4/1  "<LL_DvtComp_C>"
  [LLClb_bsLLSMConClb] -> Bus Selector3/1
  Saturation/1 -> Left Front Conner Deviation Calculation (LFCDvtCalc)/1(LFCDvtCalc_lDvt)
  Saturation1/1 -> Left Front Conner Deviation Calculation (LFCDvtCalc)/2(LFCDvtCalc_phiHdAg)
  Saturation2/1 -> Right Front Conner Deviation Calculation (RFCDvtCalc)/1(RFCDvtCalc_lDvt)
  Saturation3/1 -> Right Front Conner Deviation Calculation (RFCDvtCalc)/2(RFCDvtCalc_phiHdAg)
  Saturation4/1 -> Left Front Conner Deviation Calculation (LFCDvtCalc)/3(LFCDvtCalc_lDvtComp_C), Right Front Conner Deviation Calculation (RFCDvtCalc)/3(RFCDvtCalc_lDvtComp)

== system LKAS/LKAS/LL/LLOn/LL State Determination (LLStateDet)/LL State Machine Conditions (LLSMCon)/Activation Condition (ActvC)/Deviation Threshold Condition (DvtThresCon)/Deviation Speed Calculation (DvtSpdCalc) ==
  DvtSpdCalc_phiPrvwHdAgLft : Inport
  DvtSpdCalc_phiPrvwHdAgRgt : Inport  Port=2
  DvtSpdCalc_vVehSpd : Inport  Port=3
  Divide : Product  Inputs=**  OutDataTypeStr=single
  Divide1 : Product  Inputs=**  OutDataTypeStr=single
  Gain : Gain  Gain=1/3.6  OutDataTypeStr=single
  DvtSpdCalc_vLftDvtSpd : Outport
  DvtSpdCalc_vRgtDvtSpd : Outport  Port=2
  wires:
  Divide/1 -> DvtSpdCalc_vLftDvtSpd/1
  Divide1/1 -> DvtSpdCalc_vRgtDvtSpd/1
  DvtSpdCalc_vVehSpd/1 -> Gain/1
  Gain/1 -> Divide/2, Divide1/1
  DvtSpdCalc_phiPrvwHdAgRgt/1 -> Divide1/2
  DvtSpdCalc_phiPrvwHdAgLft/1 -> Divide/1

== system LKAS/LKAS/LL/LLOn/LL State Determination (LLStateDet)/LL State Machine Conditions (LLSMCon)/Activation Condition (ActvC)/Deviation Threshold Condition (DvtThresCon)/Deviation Threshold Judgement LDW (DvtThresJdg) ==
  DvtThresJdg_lLftDvt : Inport
  DvtThresJdg_lRgtDvt : Inport  Port=2
  DvtThresJdg_vLftDvtSpd : Inport  Port=3
  DvtThresJdg_vRgtDvtSpd : Inport  Port=4
  DvtThresJdg_tiLftTTLC : Inport  Port=5
  DvtThresJdg_tiRgtTTLC : Inport  Port=6
  DvtThresJdg_bsDvtThresClb : Inport  Port=7
  Bus Selector : BusSelector  OutputSignals=LL_DvtSpdDet_vDvtSpdMin_C
  Deviation Speed Detection (DvtSpdDet) : Subsystem
  Deviation Threshold Condition Synthesis (DTCSyn) : Subsystem
  Left Side Deviation Threshold Condition (LftDTC) : Subsystem
  Right Side Deviation Threshold Condition (RgtDTC) : Subsystem
  DvtThresJdg_stDvtThresActvFlg : Outport
  wires:
  Bus Selector/1 -> Deviation Speed Detection (DvtSpdDet)/3(DvtSpdDet_vDvtSpdMin_C)  "<LL_DvtSpdDet_vDvtSpdMin_C>"
  Deviation Speed Detection (DvtSpdDet)/1(DvtSpdDet_stDvtSpdFlg) -> Deviation Threshold Condition Synthesis (DTCSyn)/3(DTCSyn_stDvtSpdFlg)
  Deviation Threshold Condition Synthesis (DTCSyn)/1(DTCSyn_stDvtThresActvFlg) -> DvtThresJdg_stDvtThresActvFlg/1
  Right Side Deviation Threshold Condition (RgtDTC)/1(RgtDTC_stRgtDvtThresActvFlg) -> Deviation Threshold Condition Synthesis (DTCSyn)/2(DTCSyn_stRgtDvtThresActvFlg)
  Left Side Deviation Threshold Condition (LftDTC)/1(LftDTC_stLftDvtThresActvFlg) -> Deviation Threshold Condition Synthesis (DTCSyn)/1(DTCSyn_stLftDvtThresActvFlg)
  DvtThresJdg_vRgtDvtSpd/1 -> Right Side Deviation Threshold Condition (RgtDTC)/3(RgtDTC_vRgtDvtSpd), Deviation Speed Detection (DvtSpdDet)/2(DvtSpdDet_vRgtDvtSpd)
  DvtThresJdg_lRgtDvt/1 -> Right Side Deviation Threshold Condition (RgtDTC)/2(RgtDTC_lRgtDvt)
  DvtThresJdg_tiRgtTTLC/1 -> Right Side Deviation Threshold Condition (RgtDTC)/4(RgtDTC_tiRgtTTLC)
  DvtThresJdg_tiLftTTLC/1 -> Left Side Deviation Threshold Condition (LftDTC)/4(LftDTC_tiLftTTLC)
  DvtThresJdg_vLftDvtSpd/1 -> Left Side Deviation Threshold Condition (LftDTC)/3(LftDTC_vLftDvtSpd), Deviation Speed Detection (DvtSpdDet)/1(DvtSpdDet_vLftDvtSpd)
  DvtThresJdg_lLftDvt/1 -> Left Side Deviation Threshold Condition (LftDTC)/2(LftDTC_lLftDvt)
  DvtThresJdg_bsDvtThresClb/1 -> Bus Selector/1, Left Side Deviation Threshold Condition (LftDTC)/1(LftDTC_bsDvtThresInfo), Right Side Deviation Threshold Condition (RgtDTC)/1(RgtDTC_bsDvtThresInfo)

== system LKAS/LKAS/LL/LLOn/LL State Determination (LLStateDet)/LL State Machine Conditions (LLSMCon)/Activation Condition (ActvC)/Deviation Threshold Condition (DvtThresCon)/Deviation Threshold Judgement LKA (DvtThresJdg) ==
  DvtThresJdg_lLftDvt : Inport
  DvtThresJdg_lRgtDvt : Inport  Port=2
  DvtThresJdg_vLftDvtSpd : Inport  Port=3
  DvtThresJdg_vRgtDvtSpd : Inport  Port=4
  DvtThresJdg_tiLftTTLC : Inport  Port=5
  DvtThresJdg_tiRgtTTLC : Inport  Port=6
  DvtThresJdg_bsDvtThresClb : Inport  Port=7
  Bus Selector : BusSelector  OutputSignals=LL_DvtSpdDet_vDvtSpdMin_C
  Deviation Speed Detection (DvtSpdDet) : Subsystem
  Deviation Threshold Condition Synthesis (DTCSyn) : Subsystem
  Left Side Deviation Threshold Condition (LftDTC) : Subsystem
  Right Side Deviation Threshold Condition (RgtDTC) : Subsystem
  DvtThresJdg_stDvtThresActvFlg : Outport
  wires:
  DvtThresJdg_bsDvtThresClb/1 -> Right Side Deviation Threshold Condition (RgtDTC)/1(RgtDTC_bsDvtThresInfo), Left Side Deviation Threshold Condition (LftDTC)/1(LftDTC_bsDvtThresInfo), Bus Selector/1
  DvtThresJdg_lLftDvt/1 -> Left Side Deviation Threshold Condition (LftDTC)/2(LftDTC_lLftDvt)
  DvtThresJdg_vLftDvtSpd/1 -> Deviation Speed Detection (DvtSpdDet)/1(DvtSpdDet_vLftDvtSpd), Left Side Deviation Threshold Condition (LftDTC)/3(LftDTC_vLftDvtSpd)
  DvtThresJdg_tiLftTTLC/1 -> Left Side Deviation Threshold Condition (LftDTC)/4(LftDTC_tiLftTTLC)
  DvtThresJdg_tiRgtTTLC/1 -> Right Side Deviation Threshold Condition (RgtDTC)/4(RgtDTC_tiRgtTTLC)
  DvtThresJdg_lRgtDvt/1 -> Right Side Deviation Threshold Condition (RgtDTC)/2(RgtDTC_lRgtDvt)
  DvtThresJdg_vRgtDvtSpd/1 -> Deviation Speed Detection (DvtSpdDet)/2(DvtSpdDet_vRgtDvtSpd), Right Side Deviation Threshold Condition (RgtDTC)/3(RgtDTC_vRgtDvtSpd)
  Left Side Deviation Threshold Condition (LftDTC)/1(LftDTC_stLftDvtThresActvFlg) -> Deviation Threshold Condition Synthesis (DTCSyn)/1(DTCSyn_stLftDvtThresActvFlg)
  Right Side Deviation Threshold Condition (RgtDTC)/1(RgtDTC_stRgtDvtThresActvFlg) -> Deviation Threshold Condition Synthesis (DTCSyn)/2(DTCSyn_stRgtDvtThresActvFlg)
  Deviation Threshold Condition Synthesis (DTCSyn)/1(DTCSyn_stDvtThresActvFlg) -> DvtThresJdg_stDvtThresActvFlg/1
  Deviation Speed Detection (DvtSpdDet)/1(DvtSpdDet_stDvtSpdFlg) -> Deviation Threshold Condition Synthesis (DTCSyn)/3(DTCSyn_stDvtSpdFlg)
  Bus Selector/1 -> Deviation Speed Detection (DvtSpdDet)/3(DvtSpdDet_vDvtSpdMin_C)  "<LL_DvtSpdDet_vDvtSpdMin_C>"

== system LKAS/LKAS/LL/LLOn/LL State Determination (LLStateDet)/LL State Machine Conditions (LLSMCon)/Deactivation Condition (DeactvC)/Deactivation Condition Synthesis (DeactvCSyn)/Default Flag (DflFlg) ==
  Action Port : ActionPort  InitializeStates=reset  ActionType=else
  Constant : Constant  Value=0  OutDataTypeStr=boolean  SampleTime=-1
  Out : Outport
  wires:
  Constant/1 -> Out/1

== system LKAS/LKAS/LL/LLOn/LL State Determination (LLStateDet)/LL State Machine Conditions (LLSMCon)/Deactivation Condition (DeactvC)/Deactivation Condition Synthesis (DeactvCSyn)/Default Flag (DflFlg)1 ==
  Action Port : ActionPort  InitializeStates=reset  ActionType=else
  Constant : Constant  Value=0  OutDataTypeStr=boolean  SampleTime=-1
  Out : Outport
  wires:
  Constant/1 -> Out/1

== system LKAS/LKAS/LL/LLOn/LL State Determination (LLStateDet)/LL State Machine Conditions (LLSMCon)/Deactivation Condition (DeactvC)/Deactivation Condition Synthesis (DeactvCSyn)/LDW Deactivation Flag (LDWDeactvFlg) ==
  Action Port : ActionPort  InitializeStates=reset  ActionType=then
  Constant : Constant  OutDataTypeStr=boolean  SampleTime=-1
  Out : Outport
  wires:
  Constant/1 -> Out/1

== system LKAS/LKAS/LL/LLOn/LL State Determination (LLStateDet)/LL State Machine Conditions (LLSMCon)/Deactivation Condition (DeactvC)/Deactivation Condition Synthesis (DeactvCSyn)/LKA Deactivation Flag (LKADeactvFlg) ==
  Action Port : ActionPort  InitializeStates=reset  ActionType=then
  Constant : Constant  OutDataTypeStr=boolean  SampleTime=-1
  Out : Outport
  wires:
  Constant/1 -> Out/1

== system LKAS/LKAS/LL/LLOn/LL State Determination (LLStateDet)/LL State Machine Conditions (LLSMCon)/Deactivation Condition (DeactvC)/Deviation Threshold Condition (DvtThresCon)/Active Lane Calculation (ActLanCalc) ==
  ActLanCalc_bsL0Info : Inport
  ActLanCalc_bsR0Info : Inport  Port=2
  ActLanCalc_ActvCClb : Inport  Port=3
  Abs2 : Abs
  Abs3 : Abs
  Add1 : Sum
  Add2 : Sum  Inputs=+-
  Bus Creator : BusCreator  Inputs=7
  Bus Selector1 : BusSelector  OutputSignals=R0_C0
  Bus Selector2 : BusSelector  OutputSignals=L0_C0
  Bus Selector3 : BusSelector  OutputSignals=LL_ThresDet_lDvtThresLwrLDW,LL_ThresDet_lDvtThresUprLDW,LL_ThresDet_tiTTLCThresLDW,LL_ThresDet_lDvtThresLwrLKA,LL_ThresDet_lDvtThresUprLKA,LL_ThresDet_tiTTLCThresLKA,LL_DvtSpdDet_vDvtSpdMin_C
  Constant1 : Constant  Value=0.6  OutDataTypeStr=single
  Constant2 : Constant  Value=0.3  OutDataTypeStr=single
  Divide : Product  Inputs=*/
  Divide{1..6} (6 alike) : Product  Inputs=**
  Gain : Gain  Gain=0.25
  Saturation1 : Saturate  UpperLimit=5.5  LowerLimit=2.4
  Saturation2 : Saturate  UpperLimit=0.3  LowerLimit=0
  ActLanCalc_ActvCClbOut : Outport
  wires:
  Bus Selector3/7 -> Bus Creator/7  "<LL_DvtSpdDet_vDvtSpdMin_C>"
  Bus Creator/1 -> ActLanCalc_ActvCClbOut/1
  Divide6/1 -> Bus Creator/6  "LL_ThresDet_tiTTLCThresLKA"
  Divide5/1 -> Bus Creator/5  "LL_ThresDet_lDvtThresUprLKA"
  Divide4/1 -> Bus Creator/4  "LL_ThresDet_lDvtThresLwrLKA"
  Divide3/1 -> Bus Creator/3  "LL_ThresDet_tiTTLCThresLDW"
  Divide2/1 -> Bus Creator/2  "LL_ThresDet_lDvtThresUprLDW"
  Divide1/1 -> Bus Creator/1  "LL_ThresDet_lDvtThresLwrLDW"
  Divide/1 -> Divide1/1, Divide3/1, Divide4/1, Divide6/1, Divide5/1, Divide2/1
  Bus Selector3/6 -> Divide6/2  "<LL_ThresDet_tiTTLCThresLKA>"
  Bus Selector3/5 -> Divide5/2  "<LL_ThresDet_lDvtThresUprLKA>"
  Bus Selector3/4 -> Divide4/2  "<LL_ThresDet_lDvtThresLwrLKA>"
  Bus Selector3/3 -> Divide3/2  "<LL_ThresDet_tiTTLCThresLDW>"
  Saturation2/1 -> Divide/1
  Constant2/1 -> Divide/2
  Bus Selector3/2 -> Divide2/2  "<LL_ThresDet_lDvtThresUprLDW>"
  Bus Selector3/1 -> Divide1/2  "<LL_ThresDet_lDvtThresLwrLDW>"
  Add2/1 -> Saturation2/1
  Abs2/1 -> Add1/1
  Saturation1/1 -> Gain/1
  Constant1/1 -> Add2/2
  Abs3/1 -> Add1/2
  Add1/1 -> Saturation1/1
  Gain/1 -> Add2/1
  ActLanCalc_ActvCClb/1 -> Bus Selector3/1
  Bus Selector1/1 -> Abs3/1  "<R0_C0>"
  Bus Selector2/1 -> Abs2/1  "<L0_C0>"
  ActLanCalc_bsR0Info/1 -> Bus Selector1/1
  ActLanCalc_bsL0Info/1 -> Bus Selector2/1

== system LKAS/LKAS/LL/LLOn/LL State Determination (LLStateDet)/LL State Machine Conditions (LLSMCon)/Deactivation Condition (DeactvC)/Deviation Threshold Condition (DvtThresCon)/Deviation Calculation (DvtCalc) ==
  DvtCalc_bsL0Info : Inport
  DvtCalc_bsR0Info : Inport  Port=2
  Bus Selector1 : BusSelector  OutputSignals=R0_C0,R0_C1
  Bus Selector2 : BusSelector  OutputSignals=L0_C0,L0_C1
  Bus Selector3 : BusSelector  OutputSignals=EnaCClb.LL_DvtComp_C
  Left Front Conner Deviation Calculation (LFCDvtCalc) : Subsystem
  Right Front Conner Deviation Calculation (RFCDvtCalc) : Subsystem
  Saturation : Saturate  UpperLimit=3  LowerLimit=-3
  Saturation1 : Saturate  UpperLimit=0.2  LowerLimit=-0.2
  Saturation2 : Saturate  UpperLimit=3  LowerLimit=-3
  Saturation3 : Saturate  UpperLimit=0.2  LowerLimit=-0.2
  Saturation4 : Saturate  UpperLimit=0.1  LowerLimit=-0.1
  DvtCalc_lLftDvt : Outport
  DvtCalc_lRgtDvt : Outport  Port=2
  wires:
  DvtCalc_bsL0Info/1 -> Bus Selector2/1
  DvtCalc_bsR0Info/1 -> Bus Selector1/1
  Left Front Conner Deviation Calculation (LFCDvtCalc)/1(DvtCalc_lLftDvt) -> DvtCalc_lLftDvt/1
  Right Front Conner Deviation Calculation (RFCDvtCalc)/1(DvtCalc_lRgtDvt) -> DvtCalc_lRgtDvt/1
  Bus Selector2/1 -> Saturation/1  "<L0_C0>"
  Bus Selector2/2 -> Saturation1/1  "<L0_C1>"
  Bus Selector1/1 -> Saturation2/1  "<R0_C0>"
  Bus Selector1/2 -> Saturation3/1  "<R0_C1>"
  Bus Selector3/1 -> Saturation4/1  "<LL_DvtComp_C>"
  [LLClb_bsLLSMConClb] -> Bus Selector3/1
  Saturation/1 -> Left Front Conner Deviation Calculation (LFCDvtCalc)/1(LFCDvtCalc_lDvt)
  Saturation1/1 -> Left Front Conner Deviation Calculation (LFCDvtCalc)/2(LFCDvtCalc_phiHdAg)
  Saturation2/1 -> Right Front Conner Deviation Calculation (RFCDvtCalc)/1(RFCDvtCalc_lDvt)
  Saturation3/1 -> Right Front Conner Deviation Calculation (RFCDvtCalc)/2(RFCDvtCalc_phiHdAg)
  Saturation4/1 -> Right Front Conner Deviation Calculation (RFCDvtCalc)/3(RFCDvtCalc_lDvtComp), Left Front Conner Deviation Calculation (LFCDvtCalc)/3(LFCDvtCalc_lDvtComp_C)

== system LKAS/LKAS/LL/LLOn/LL State Determination (LLStateDet)/LL State Machine Conditions (LLSMCon)/Deactivation Condition (DeactvC)/Deviation Threshold Condition (DvtThresCon)/Deviation Speed Calculation (DvtSpdCalc) ==
  DvtSpdCalc_phiPrvwHdAgLft : Inport
  DvtSpdCalc_phiPrvwHdAgRgt : Inport  Port=2
  DvtSpdCalc_vVehSpd : Inport  Port=3
  Divide : Product  Inputs=**  OutDataTypeStr=single
  Divide1 : Product  Inputs=**  OutDataTypeStr=single
  Gain : Gain  Gain=1/3.6  OutDataTypeStr=single
  DvtSpdCalc_vLftDvtSpd : Outport
  DvtSpdCalc_vRgtDvtSpd : Outport  Port=2
  wires:
  Divide/1 -> DvtSpdCalc_vLftDvtSpd/1
  Divide1/1 -> DvtSpdCalc_vRgtDvtSpd/1
  DvtSpdCalc_vVehSpd/1 -> Gain/1
  Gain/1 -> Divide/2, Divide1/1
  DvtSpdCalc_phiPrvwHdAgRgt/1 -> Divide1/2
  DvtSpdCalc_phiPrvwHdAgLft/1 -> Divide/1

== system LKAS/LKAS/LL/LLOn/LL State Determination (LLStateDet)/LL State Machine Conditions (LLSMCon)/Deactivation Condition (DeactvC)/Deviation Threshold Condition (DvtThresCon)/Deviation Threshold Judgement LDW (DvtThresJdg) ==
  DvtThresJdg_lLftDvt : Inport
  DvtThresJdg_lRgtDvt : Inport  Port=2
  DvtThresJdg_vLftDvtSpd : Inport  Port=3
  DvtThresJdg_vRgtDvtSpd : Inport  Port=4
  DvtThresJdg_tiLftTTLC : Inport  Port=5
  DvtThresJdg_tiRgtTTLC : Inport  Port=6
  DvtThresJdg_bsDvtThresClb : Inport  Port=7
  Bus Selector : BusSelector  OutputSignals=LL_DvtSpdDet_vDvtSpdMin_C
  Deviation Speed Detection (DvtSpdDet) : Subsystem
  Deviation Threshold Condition Synthesis (DTCSyn) : Subsystem
  Left Side Deviation Threshold Condition (LftDTC) : Subsystem
  Right Side Deviation Threshold Condition (RgtDTC) : Subsystem
  DvtThresJdg_stDvtThresActvFlg : Outport
  wires:
  Bus Selector/1 -> Deviation Speed Detection (DvtSpdDet)/3(DvtSpdDet_vDvtSpdMin_C)  "<LL_DvtSpdDet_vDvtSpdMin_C>"
  Deviation Speed Detection (DvtSpdDet)/1(DvtSpdDet_stDvtSpdFlg) -> Deviation Threshold Condition Synthesis (DTCSyn)/3(DTCSyn_stDvtSpdFlg)
  Deviation Threshold Condition Synthesis (DTCSyn)/1(DTCSyn_stDvtThresActvFlg) -> DvtThresJdg_stDvtThresActvFlg/1
  Right Side Deviation Threshold Condition (RgtDTC)/1(RgtDTC_stRgtDvtThresActvFlg) -> Deviation Threshold Condition Synthesis (DTCSyn)/2(DTCSyn_stRgtDvtThresActvFlg)
  Left Side Deviation Threshold Condition (LftDTC)/1(LftDTC_stLftDvtThresActvFlg) -> Deviation Threshold Condition Synthesis (DTCSyn)/1(DTCSyn_stLftDvtThresActvFlg)
  DvtThresJdg_vRgtDvtSpd/1 -> Right Side Deviation Threshold Condition (RgtDTC)/3(RgtDTC_vRgtDvtSpd), Deviation Speed Detection (DvtSpdDet)/2(DvtSpdDet_vRgtDvtSpd)
  DvtThresJdg_lRgtDvt/1 -> Right Side Deviation Threshold Condition (RgtDTC)/2(RgtDTC_lRgtDvt)
  DvtThresJdg_tiRgtTTLC/1 -> Right Side Deviation Threshold Condition (RgtDTC)/4(RgtDTC_tiRgtTTLC)
  DvtThresJdg_tiLftTTLC/1 -> Left Side Deviation Threshold Condition (LftDTC)/4(LftDTC_tiLftTTLC)
  DvtThresJdg_vLftDvtSpd/1 -> Left Side Deviation Threshold Condition (LftDTC)/3(LftDTC_vLftDvtSpd), Deviation Speed Detection (DvtSpdDet)/1(DvtSpdDet_vLftDvtSpd)
  DvtThresJdg_lLftDvt/1 -> Left Side Deviation Threshold Condition (LftDTC)/2(LftDTC_lLftDvt)
  DvtThresJdg_bsDvtThresClb/1 -> Bus Selector/1, Left Side Deviation Threshold Condition (LftDTC)/1(LftDTC_bsDvtThresInfo), Right Side Deviation Threshold Condition (RgtDTC)/1(RgtDTC_bsDvtThresInfo)
